simulink model "HCS_Sim_r9_final"  (R2023a)
settings: Solver=ode4  StartTime=0.0  StopTime=24  FixedStep=5e-3  RelTol=1e-3  EnableMultiTasking=on
libraries: simulink x26, simulink_extras x11, arduinolib x8, spspowerguiLib x1
(part 1 of 5)
settings Model: ExtModeTrigDuration=2  Creator=jakob  LastModifiedBy=Matt Smith
settings OptimizationCC: EnhancedBackFolding=on  PassReuseOutputArgsAs=Individual arguments  ZeroExternalMemoryAtStartup=off  ZeroInternalMemoryAtStartup=off  MaxStackSize=64  OptimizeBlockOrder=speed  DifferentSizesBufferReuse=on  OptimizationCustomize=off  EfficientTunableParamExpr=on
settings DebuggingCC: ParameterTunabilityLossMsg=error  UnderSpecifiedDimensionMsg=warning
settings HardwareCC: ProdBitPerInt=16  ProdBitPerPointer=16  ProdBitPerSizeT=16  ProdBitPerPtrDiffT=16  ProdLargestAtomicFloat=None  ProdWordSize=8  ProdHWDeviceType=Atmel->AVR
settings SFSimCC: MATLABDynamicMemAlloc=off  SimTargetLang=C++
settings RTWCC: Description=Embedded Coder  SystemTargetFile=ert.tlc  HardwareBoard=Arduino Uno  TemplateMakefile=ert_default_tmf  Toolchain=Arduino AVR  BuildConfiguration=Faster Runs
settings CodeAppCC: ForceParamTrailComments=on  IgnoreCustomStorageClasses=off  OperatorAnnotations=on  SimulinkDataObjDesc=on  SFDataObjDesc=on  InsertBlockDesc=on
settings ERTTargetCC: SupportContinuousTime=on  SupportVariableSizeSignals=on  ExtModeTransport=3  ExtModeStaticAlloc=on  ExtModeAutomaticAllocSize=off  ExtModeStaticAllocSize=250  ExtModeMexFile=ext_xcp  ExtModeIntrfLevel=Level2 - Open

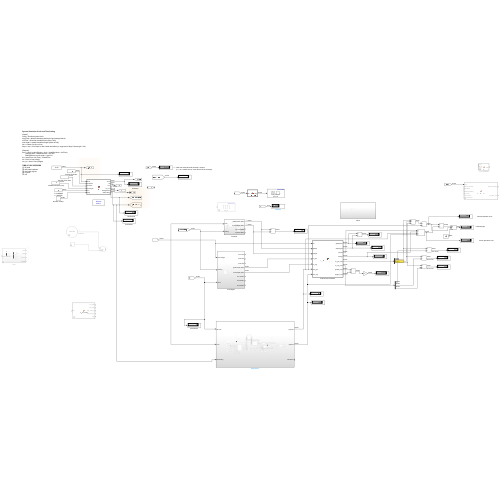
[thumbnail: Simulink's stored preview of the top-level diagram]
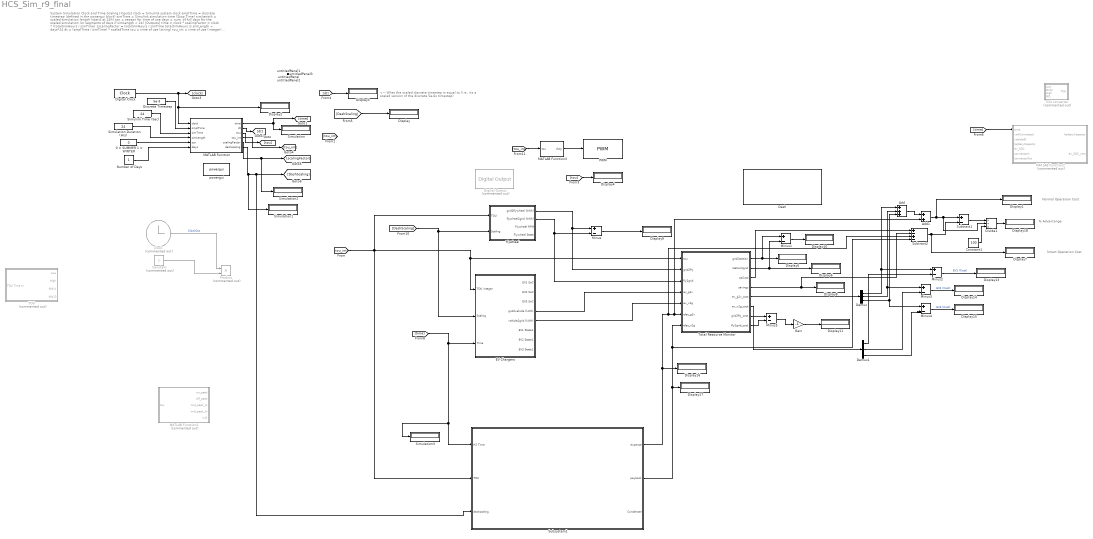
== system HCS_Sim_r9_final ==
  note: Smart Operation Cost
  note: % Advantange
  note: Normal Operation Cost
  note: <--- What the scaled discrete timestep is equal to
      | 	(i.e., its a scaled version of the discrete 5e-6s timestep)
  note: System Simulation Clock and Time Scaling
      |
      | [Inputs]
      | clock = Simulink system clock
      | smplTime = discrete timestep (defined in the powergui block)
      | simTime = Simulink simulation time (Stop Time)
      | simLength = scaled simulation length (static at 24h)
      | szn = season for time of use
      | days = num. of full days for the scaled simulation (or segments of days if simLength < 24)
      |
      | [Outputs]
      | time = clock * scalingFactor = clock * (totalSimHours / simTime)
      | {scalingFactor = totalSimHours / simTime
      | totalSimHours is simLength + days*24
      | dt = (smplTime / simTime) * scaledTime
      | tou = time of use (string)
      | tou_int = time of use (integer)
      |
      | TIME OF USE INTEGERS
      | [1] off peak
      | [2] mid peak low/down
      | [3] mid peak high/up
      | [4] on peak
      | [5] null
  0 = SUMMER 1 = WINTER : Constant  Value=0
  Add : Sum  Inputs=+++
  Add1 : Sum
  Clock : Clock  Commented=on
  Constant : Constant  Commented=on
  Constant1 : Constant  Value=100
  Dash : Subsystem
  Demux : Demux  Outputs=3
  Demux1 : Demux  Outputs=3
  Digital Clock : DigitalClock  SampleTime=5e-3
  Digital Output : arduinolib/Digital Output  Commented=on  pinNumber=9  Direction=output  blockPlatform=arduino
  Discrete Timestep : Constant  Value=5e-3
  Display{,1..11,13..18} (18 alike) : Display
  Divide1 : Product  Inputs=*/*
  EV Chargers : Subsystem
  Flywheel : Subsystem  StopFcn=CapTest
  Gain : Gain  Gain=-1
  MATLAB Function : MATLAB Function  TreatAsAtomicUnit=on
  MATLAB Function1 : MATLAB Function  Commented=on  TreatAsAtomicUnit=on
  MATLAB Function2 : MATLAB Function  Commented=on  TreatAsAtomicUnit=on
  MATLAB Function3 : MATLAB Function  TreatAsAtomicUnit=on
  Minus{,1..5} (6 alike) : Sum  Inputs=+-
  Number of Days : Constant
  PWM : arduinolib/PWM  pinNumber=10  frequencyType=Default  desiredFrequency=490.2  achievableFrequency=490.1961
  Product : Product  Commented=on
  Simulation{,1..3} (4 alike) : Display
  Simulation Duration (Hrs) : Constant  Value=24
  Simulink Time (Sec) : Constant  Value=24
  Subsystem1 : Subsystem
  Subtract1 : Sum  Inputs=+-
  Subtract2 : Sum  Inputs=+-+-
  TOU : Subsystem  Commented=on
  TOU converter : MATLAB Function  Commented=on  TreatAsAtomicUnit=on
  Total Resource Monitor : MATLAB Function  TreatAsAtomicUnit=on
  powergui : spspowerguiLib/powergui  Priority=1  SimulationMode=Discrete  SampleTime=5e-3  frequency=60  Iterations=50  frequencyindice=0  Pbase=100e6  ErrMax=1e-4  UnitsV=kV  UnitsW=MW  buscounter=0  FunctionMessages=off  echomessages=off  EnableUseOfTLC=off  CurrentSourceSwitches=off  DisableSnubberDevices=off  DisableRonSwitches=off  DisableVfSwitches=off  DisplayEquations=off  AutomaticDiscreteSolvers=off  SolverType=Tustin/Backward Euler (TBE)  Interpol=off  ExternalGateDelay=off  methode=off  Ts=100  x0status=blocks  SPID=on  SwTol=0  HookPort=off  NonlinearTolerance=1e-4  nMaxIteration=100  ContinueOnMaxIteration=off  RestoreLinks=warning  ResistiveCurrentMeasurement=off  Frange=[0:2:500]  Ylog=off  Xlog=on  ShowGrid=off  save=off  variable=ZData  structure=0  ZoomFFT=off  StartTime=0.0  cycles=1  DisplayStyle=1  fundamental=60  FreqAxis=off  MaxFrequency=1000  frequencyindicesteady=1  RmsSteady=1  display=off
  untitledPanel : Subsystem  Tag=HiddenForWebPanel  IsWebBlockPanel=on
  untitledPanel1 : Subsystem  Tag=HiddenForWebPanel  IsWebBlockPanel=on
  untitledPanel2 : Subsystem  Tag=HiddenForWebPanel  IsWebBlockPanel=on
  untitledPanel3 : Subsystem  Tag=HiddenForWebPanel  IsWebBlockPanel=on
  wires:
  Clock/1 -> Product/1  "ClockOut"
  Constant/1 -> Product/2
  MATLAB Function/1(time) -> [time], Simulation/1
  MATLAB Function/3(tou) -> [tou]
  Digital Clock/1 -> [clock], MATLAB Function/1(clock), Display2/1
  Number of Days/1 -> MATLAB Function/6(days)
  Discrete Timestep/1 -> MATLAB Function/2(smplTime)
  Simulink Time (Sec)/1 -> MATLAB Function/3(simTime)
  Simulation Duration (Hrs)/1 -> MATLAB Function/4(simLength)
  MATLAB Function/4(tou_int) -> [tou_int]
  MATLAB Function/2(dt) -> [dt]
  0 = SUMMER 1 = WINTER/1 -> MATLAB Function/5(szn)
  [tou] -> Display4/1
  [dt] -> Display3/1
  MATLAB Function/5(scalingFactor) -> Simulation2/1, [scalingFactor]
  [tou_int] -> Subsystem1/2(TOU), EV Chargers/1(TOU integer), Total Resource Monitor/1(tou), Flywheel/1(TOU)
  [time] -> MATLAB Function2/1(time)
  MATLAB Function/6(dashscaling) -> Simulation1/1, Subsystem1/3(dashscaling), [DashScaling]
  [DashScaling] -> Display/1
  [tou_int] -> MATLAB Function3/1(tou)
  MATLAB Function3/1(duty) -> PWM/1
  [DashScaling] -> Flywheel/2(Scaling), EV Chargers/2(Scaling)
  Flywheel/1(grid2flywheel (kWh)) -> Total Resource Monitor/2(grid2fly), Minus/1
  Flywheel/2(flywheel2grid (kWh)) -> Total Resource Monitor/3(fly2grid), Minus/2
  Total Resource Monitor/1(grid2station) -> Minus1/1, Display5/1
  Total Resource Monitor/2(station2grid) -> Minus1/2, Display6/1
  Total Resource Monitor/3(opCost) -> Subtract2/1
  Total Resource Monitor/4(savings) -> Subtract2/2, Display8/1
  Total Resource Monitor/5(ev_g2v_cost) -> Demux/1
  [time] -> Subsystem1/1(H2 Time), Simulation3/1, EV Chargers/3(Time)
  Total Resource Monitor/7(grid2fly_cost) -> Minus5/1
  Total Resource Monitor/8(fly2grid_cost) -> Minus5/2
  EV Chargers/4(grid2vehicle (kWh)) -> Total Resource Monitor/4(ev_g2v)
  EV Chargers/5(vehicle2grid (kWh)) -> Total Resource Monitor/5(ev_v2g)
  Demux1/3 -> Minus4/2
  Total Resource Monitor/6(ev_v2g_cost) -> Demux1/1
  Demux1/2 -> Minus3/2
  Demux1/1 -> Minus2/2
  Demux/3 -> Minus4/1, Add/3
  Demux/2 -> Add/2, Minus3/1
  Demux/1 -> Add/1, Minus2/1
  Minus/1 -> Display9/1
  Minus1/1 -> Display10/1
  Minus2/1 -> Display13/1  "EV1 (Cost)"
  Minus3/1 -> Display14/1  "EV2 (Cost)"
  Minus4/1 -> Display15/1  "EV3 (Cost)"
  Minus5/1 -> Gain/1
  Gain/1 -> Display11/1
  Subsystem1/2(payback) -> Display17/1, Subtract2/4, Total Resource Monitor/7(elec_v2g)
  Subsystem1/1(expense) -> Display16/1, Subtract2/3, Add1/2, Total Resource Monitor/6(elec_g2v)
  Add/1 -> Add1/1
  Add1/1 -> Display1/1, Divide1/2, Subtract1/1
  Subtract2/1 -> Display7/1, Subtract1/2
  Subtract1/1 -> Divide1/1
  Divide1/1 -> Display18/1
  Constant1/1 -> Divide1/3

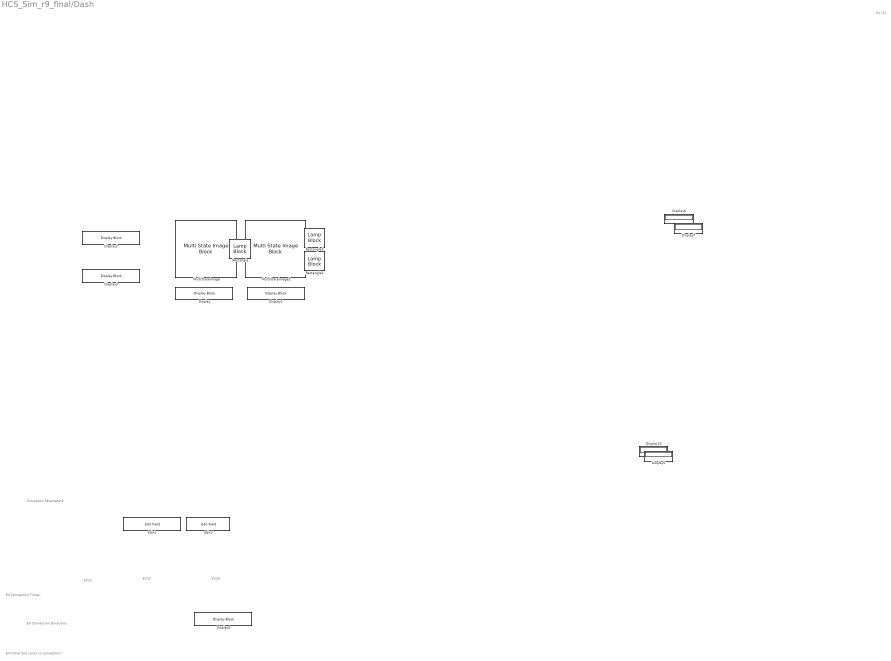
== system HCS_Sim_r9_final/Dash ==
  note: EV (2)
  note: EV Connection Times:
  note: EV Connection
      | Durations:
  note: EV Initial SoC (prior
      | to connection):
  note: EV(1)
  note: EV(2)
  note: EV(3)
  note: Simulation Parameters:
  Display{,1..4} (5 alike) : DisplayBlock  LabelPosition=Hide  Transparency=1
      Display2 settings: AttributesFormatString=Hydrogen Output (KG)
      Display3 settings: AttributesFormatString=FCEVs Fueled
  Display{5..7,16} (4 alike) : Display
  Edit1 : EditField  LabelPosition=Bottom  ShowInitialText=on  Alignment=Center
  Edit2 : EditField  LabelPosition=Bottom  ShowInitialText=on  Alignment=Center
  MultiStateImage : MultiStateImageBlock  Description=10KG pressurized 700Bar
      settings: AttributesFormatString=10KG pressurized 700Bar
  MultiStateImage1 : MultiStateImageBlock
      settings: AttributesFormatString=10KG pressurized 200Bar
  Rectangle : LampBlock  LabelPosition=Hide  Icon=Rectangle
      settings: AttributesFormatString=Compressor
  Rectangle2 : LampBlock  LabelPosition=Hide  Icon=Rectangle
      settings: AttributesFormatString=Reverse Electrolysis
  Rectangle3 : LampBlock  LabelPosition=Hide  Icon=Rectangle
      settings: AttributesFormatString=Electrolysis

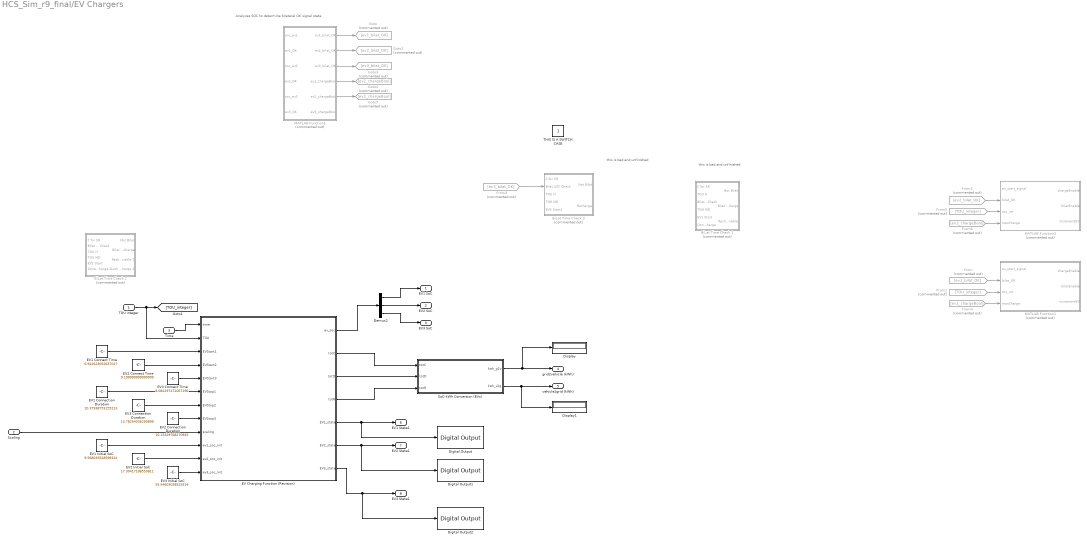
== system HCS_Sim_r9_final/EV Chargers ==
  note: this is bad and unfinished
  note: Analyzes SOC to determine bilateral OK signal state
  note: this is bad and unfinished
  TOU integer : Inport
  Scaling : Inport  Port=2
  Time : Inport  Port=3
  BiLat Time Check 1 : Subsystem  Commented=on
  BiLat Time Check 2 : Subsystem  Commented=on
  BiLat Time Check 3 : Subsystem  Commented=on
  Demux2 : Demux  Outputs=3
  Digital Output : arduinolib/Digital Output  pinNumber=6  Direction=output  blockPlatform=arduino
  Digital Output1 : arduinolib/Digital Output  pinNumber=7  Direction=output  blockPlatform=arduino
  Digital Output2 : arduinolib/Digital Output  pinNumber=8  Direction=output  blockPlatform=arduino
  Display : Display
  Display1 : Display
  EV Charging Function (Revision) : MATLAB Function  TreatAsAtomicUnit=on
  EV1 Connect Time : Constant  Value=6.922623052637027
  EV1 Connection Duration : Constant  Value=10.37938753155213
  EV1 Initial SoC : Constant  Value=9.568033528599324
  EV2 Connect Time : Constant  Value=9.199999999999999
  EV2 Connection Duration : Constant  Value=10.15329768270945
  EV2 Initial SoC : Constant  Value=17.30417188553811
  EV3 Connect Time : Constant  Value=8.082297471067296
  EV3 Connection Duration : Constant  Value=13.78254036290899
  EV3 Initial SoC : Constant  Value=55.54603038529314
  From : From  Commented=on  GotoTag=ev1_bilat_OK
  From1 : From  Commented=on  GotoTag=TOU_integer
  From2 : From  Commented=on  GotoTag=ev2_bilat_OK
  From3 : From  Commented=on  GotoTag=ev3_bilat_OK
  From4 : From  Commented=on  GotoTag=ev1_chargeBool
  From5 : From  Commented=on  GotoTag=TOU_integer
  From6 : From  Commented=on  GotoTag=ev2_chargeBool
  Goto : Goto  Commented=on  GotoTag=ev1_bilat_OK
  Goto2 : Goto  Commented=on  GotoTag=ev2_bilat_OK
  Goto3 : Goto  Commented=on  GotoTag=ev3_bilat_OK
  Goto4 : Goto  Commented=on  GotoTag=ev1_chargeBool
  Goto5 : Goto  Commented=on  GotoTag=ev2_chargeBool
  MATLAB Function1 : MATLAB Function  Commented=on  TreatAsAtomicUnit=on
  MATLAB Function2 : MATLAB Function  Commented=on  TreatAsAtomicUnit=on
  MATLAB Function3 : MATLAB Function  Commented=on  TreatAsAtomicUnit=on
  SoC-kWh Conversion (EVs) : MATLAB Function  TreatAsAtomicUnit=on
  THIS IS A SWITCH CASE : Constant
  EV1 SoC : Outport
  EV2 SoC : Outport  Port=2
  EV3 SoC : Outport  Port=3
  grid2vehicle (kWh) : Outport  Port=4
  vehicle2grid (kWh) : Outport  Port=5
  EV1 State1 : Outport  Port=6
  EV2 State1 : Outport  Port=7
  EV3 State1 : Outport  Port=8
  wires:
  MATLAB Function1/1(ev1_bilat_OK) -> Goto/1
  MATLAB Function1/2(ev2_bilat_OK) -> Goto2/1
  MATLAB Function1/3(ev3_bilat_OK) -> Goto3/1
  From/1 -> MATLAB Function2/2(bilat_OK)
  From1/1 -> MATLAB Function2/3(tou_int)
  From3/1 -> BiLat Time Check 3/2(Bilat SOC Check)
  MATLAB Function1/4(ev1_chargeBool) -> Goto4/1
  From4/1 -> MATLAB Function2/4(maxCharge)
  From2/1 -> MATLAB Function3/2(bilat_OK)
  From5/1 -> MATLAB Function3/3(tou_int)
  From6/1 -> MATLAB Function3/4(maxCharge)
  MATLAB Function1/5(ev2_chargeBool) -> Goto5/1
  Scaling/1 -> EV Charging Function (Revision)/9(scaling)
  TOU integer/1 -> EV Charging Function (Revision)/2(TOU), [TOU_integer]
  SoC-kWh Conversion (EVs)/1(kwh_g2v) -> Display/1, grid2vehicle (kWh)/1
  SoC-kWh Conversion (EVs)/2(kwh_v2g) -> Display1/1, vehicle2grid (kWh)/1
  Time/1 -> EV Charging Function (Revision)/1(time)
  EV3 Connect Time/1 -> EV Charging Function (Revision)/5(EVStart3)
  EV2 Connect Time/1 -> EV Charging Function (Revision)/4(EVStart2)
  EV1 Connect Time/1 -> EV Charging Function (Revision)/3(EVStart1)
  EV2 Connection Duration/1 -> EV Charging Function (Revision)/8(EVStop3)
  EV3 Connection Duration/1 -> EV Charging Function (Revision)/7(EVStop2)
  EV1 Connection Duration/1 -> EV Charging Function (Revision)/6(EVStop1)
  EV Charging Function (Revision)/1(ev_soc) -> Demux2/1
  Demux2/1 -> EV1 SoC/1
  Demux2/2 -> EV2 SoC/1
  Demux2/3 -> EV3 SoC/1
  EV Charging Function (Revision)/2(totC) -> SoC-kWh Conversion (EVs)/1(totC)
  EV Charging Function (Revision)/3(totD) -> SoC-kWh Conversion (EVs)/2(totD)
  EV Charging Function (Revision)/4(totR) -> SoC-kWh Conversion (EVs)/3(totR)
  EV Charging Function (Revision)/5(EV1_state) -> Digital Output/1, EV1 State1/1
  EV Charging Function (Revision)/6(EV2_state) -> Digital Output1/1, EV2 State1/1
  EV Charging Function (Revision)/7(EV3_state) -> Digital Output2/1, EV3 State1/1
  EV1 Initial SoC/1 -> EV Charging Function (Revision)/10(ev1_soc_init)
  EV2 Initial SoC/1 -> EV Charging Function (Revision)/11(ev2_soc_init)
  EV3 Initial SoC/1 -> EV Charging Function (Revision)/12(ev3_soc_init)

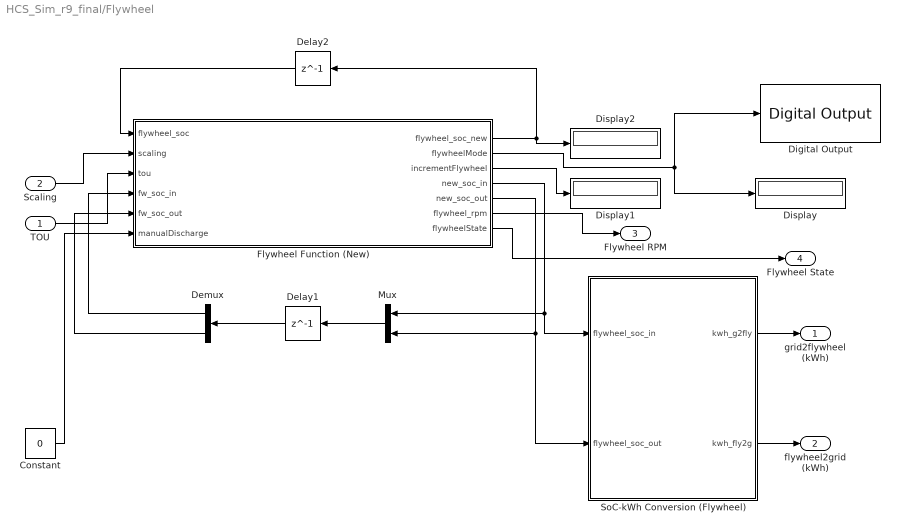
== system HCS_Sim_r9_final/Flywheel ==
  TOU : Inport
  Scaling : Inport  Port=2
  Constant : Constant  Value=0
  Delay1 : Delay  DelayLength=1
  Delay2 : Delay  DelayLength=1
  Demux : Demux  Outputs=2
  Digital Output : arduinolib/Digital Output  pinNumber=5  Direction=output  blockPlatform=arduino
  Display : Display
      settings: Decimation=4
  Display1 : Display
      settings: Decimation=4
  Display2 : Display
      settings: Decimation=4
  Flywheel Function (New) : MATLAB Function  TreatAsAtomicUnit=on
  Mux : Mux  Inputs=2
  SoC-kWh Conversion (Flywheel) : MATLAB Function  TreatAsAtomicUnit=on
  grid2flywheel (kWh) : Outport
  flywheel2grid (kWh) : Outport  Port=2
  Flywheel RPM : Outport  Port=3
  Flywheel State : Outport  Port=4
  wires:
  Flywheel Function (New)/1(flywheel_soc_new) -> Delay2/1, Display2/1
  Delay2/1 -> Flywheel Function (New)/1(flywheel_soc)
  Scaling/1 -> Flywheel Function (New)/2(scaling)
  TOU/1 -> Flywheel Function (New)/3(tou)
  Flywheel Function (New)/3(incrementFlywheel) -> Display1/1
  Flywheel Function (New)/2(flywheelMode) -> Display/1, Digital Output/1
  SoC-kWh Conversion (Flywheel)/1(kwh_g2fly) -> grid2flywheel (kWh)/1
  SoC-kWh Conversion (Flywheel)/2(kwh_fly2g) -> flywheel2grid (kWh)/1
  Mux/1 -> Delay1/1
  Flywheel Function (New)/4(new_soc_in) -> SoC-kWh Conversion (Flywheel)/1(flywheel_soc_in), Mux/1
  Flywheel Function (New)/5(new_soc_out) -> Mux/2, SoC-kWh Conversion (Flywheel)/2(flywheel_soc_out)
  Delay1/1 -> Demux/1
  Demux/1 -> Flywheel Function (New)/4(fw_soc_in)
  Demux/2 -> Flywheel Function (New)/5(fw_soc_out)
  Flywheel Function (New)/6(flywheel_rpm) -> Flywheel RPM/1
  Flywheel Function (New)/7(flywheelState) -> Flywheel State/1
  Constant/1 -> Flywheel Function (New)/6(manualDischarge)

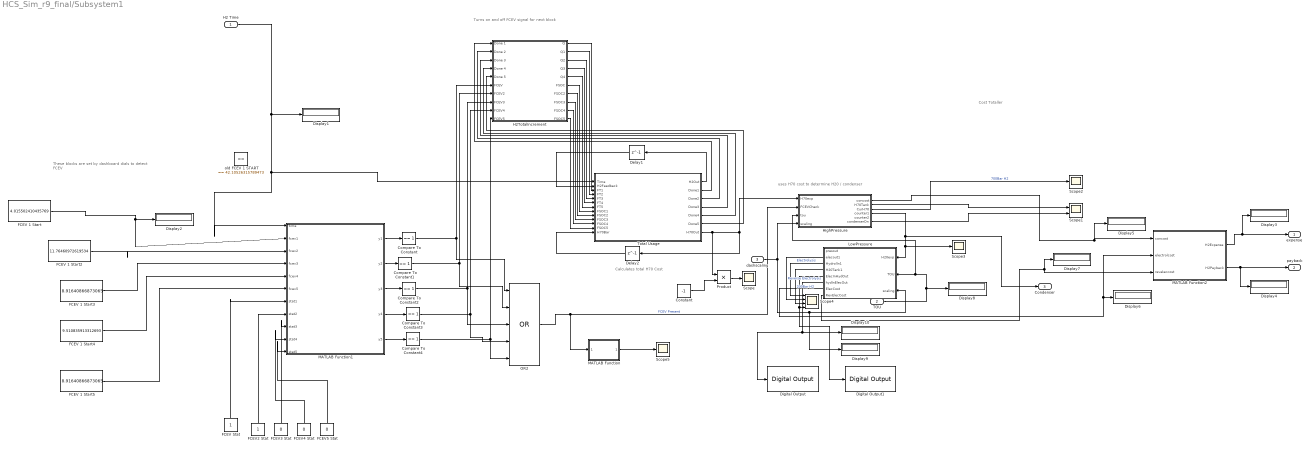
== system HCS_Sim_r9_final/Subsystem1 ==
  note: uses H70 cost to determine H20 / condenser
  note: Calculates total H70 Cost
  note: Turns on and off FCEV signal for next block
  note: These blocks are set by dashboard dials to detect FCEV
  note: Cost Totaller
  H2 Time : Inport
  TOU : Inport  Port=2
  dashscaling : Inport  Port=3
  Compare To Constant{,1..4} (5 alike) : simulink/Logic and Bit Operations/Compare To Constant  relop===  const=1  OutDataTypeStr=boolean
  Constant : Constant  Value=-1
  Delay1 : Delay  DelayLength=1  InitialCondition=0
  Delay2 : Delay  DelayLength=1  InitialCondition=0
  Digital Output : arduinolib/Digital Output  pinNumber=4  Direction=output  blockPlatform=arduino
  Digital Output1 : arduinolib/Digital Output  pinNumber=3  Direction=output  blockPlatform=arduino
  Display{1..10} (10 alike) : Display
  FCEV 1 Start : Constant  Value=4.015502410435769
  FCEV 1 Start2 : Constant  Value=11.76460972619534
  FCEV 1 Start3 : Constant  Value=8.91640866873065
  FCEV 1 Start4 : Constant  Value=9.510835913312693
  FCEV 1 Start5 : Constant  Value=8.91640866873065
  FCEV Stat : Constant
  FCEV2 Stat : Constant
  FCEV3 Stat : Constant  Value=0
  FCEV4 Stat : Constant  Value=0
  FCEV5 Stat : Constant  Value=0
  H2TotalIncrement : Subsystem
  HighPressure : MATLAB Function  TreatAsAtomicUnit=on
  LowPressure : MATLAB Function  TreatAsAtomicUnit=on
  MATLAB Function : MATLAB Function  TreatAsAtomicUnit=on
  MATLAB Function1 : MATLAB Function  TreatAsAtomicUnit=on
  MATLAB Function2 : MATLAB Function  TreatAsAtomicUnit=on
  OR2 : Logic  Operator=OR  Inputs=5  IconShape=distinctive  AllPortsSameDT=off  OutDataTypeStr=boolean
  Product : Product
  Scope{,2..3,5} (4 alike) : Scope
  Scope1 : Scope  NumInputPorts=2
  Scope4 : Scope  NumInputPorts=4
  Total Usage : MATLAB Function  TreatAsAtomicUnit=on
  old FCEV 1 START : simulink/Logic and Bit Operations/Compare To Constant  relop===  const=42.10526315789473  OutDataTypeStr=boolean
  expense : Outport
  payback : Outport  Port=2
  Condenser : Outport  Port=3
  wires:
  MATLAB Function1/1(y1) -> Compare To Constant/1
  OR2/1 -> MATLAB Function/1(FCEVIn), HighPressure/2(FCEVCheck)  "FCEV Present"
  MATLAB Function1/3(y3) -> Compare To Constant2/1
  MATLAB Function1/2(y2) -> Compare To Constant1/1
  Total Usage/1(H2Out) -> Delay1/1
  MATLAB Function1/4(y4) -> Compare To Constant3/1
  MATLAB Function1/5(y5) -> Compare To Constant4/1
  Total Usage/2(Done1) -> H2TotalIncrement/1(Done 1)
  Total Usage/3(Done2) -> H2TotalIncrement/2(Done 2)
  Total Usage/4(Done3) -> H2TotalIncrement/3(Done 3)
  Total Usage/5(Done4) -> H2TotalIncrement/4(Done 4)
  Total Usage/6(Done5) -> H2TotalIncrement/5(Done 5)
  Total Usage/7(H70Out) -> Product/1, Delay2/1, HighPressure/1(H70exp)
  H2TotalIncrement/1(Q) -> Total Usage/3(FT1)
  H2TotalIncrement/2(Q1) -> Total Usage/4(FT2)
  H2TotalIncrement/3(Q2) -> Total Usage/5(FT3)
  H2TotalIncrement/4(Q3) -> Total Usage/6(FT4)
  H2TotalIncrement/5(Q4) -> Total Usage/7(FT5)
  Delay2/1 -> Total Usage/13(H70Bar)
  H2TotalIncrement/6(FSOC) -> Total Usage/8(FSOC1)
  H2TotalIncrement/7(FSOC2) -> Total Usage/9(FSOC2)
  H2TotalIncrement/8(FSOC3) -> Total Usage/10(FSOC3)
  H2TotalIncrement/9(FSOC4) -> Total Usage/11(FSOC4)
  H2TotalIncrement/10(FSOC5) -> Total Usage/12(FSOC5)
  Delay1/1 -> Total Usage/2(H2Feedback)
  HighPressure/2(H70Tank) -> Scope1/1
  HighPressure/3(CurH70) -> Scope2/1  "700Bar H2"
  HighPressure/4(counter1) -> Condenser/1, LowPressure/1(H20exp), Scope3/1
  TOU/1 -> Display8/1, HighPressure/3(tou), LowPressure/2(TOU)
  LowPressure/3(HydrolIn1) -> Scope4/1  "Electrolysis"
  LowPressure/2(elecout1) -> Scope4/2  "Reverse Electrolysis"
  LowPressure/4(H20Tank1) -> Scope4/3  "200Bar H2"
  LowPressure/5(ElecInHydOut) -> Digital Output1/1, Scope4/4
  HighPressure/6(condenserOn) -> Scope1/2
  MATLAB Function/1(FCEVPres) -> Scope5/1
  FCEV 1 Start/1 -> MATLAB Function1/2(fcev1), Display2/1
  FCEV Stat/1 -> MATLAB Function1/7(stat1)
  FCEV2 Stat/1 -> MATLAB Function1/8(stat2)
  FCEV3 Stat/1 -> MATLAB Function1/9(stat3)
  FCEV4 Stat/1 -> MATLAB Function1/10(stat4)
  FCEV5 Stat/1 -> MATLAB Function1/11(stat5)
  FCEV 1 Start5/1 -> MATLAB Function1/6(fcev5)
  FCEV 1 Start4/1 -> MATLAB Function1/5(fcev4)
  FCEV 1 Start3/1 -> MATLAB Function1/4(fcev3)
  FCEV 1 Start2/1 -> MATLAB Function1/3(fcev2)
  Compare To Constant/1 -> H2TotalIncrement/6(FCEV), OR2/1
  Compare To Constant1/1 -> H2TotalIncrement/7(FCEV2), OR2/2
  Compare To Constant2/1 -> H2TotalIncrement/8(FCEV3), OR2/3
  Compare To Constant3/1 -> H2TotalIncrement/9(FCEV4), OR2/4
  Compare To Constant4/1 -> H2TotalIncrement/10(FCEV5), OR2/5
  H2 Time/1 -> Display1/1, MATLAB Function1/1(time), Total Usage/1(Time)
  Constant/1 -> Product/2
  Product/1 -> Scope/1
  HighPressure/1(concost) -> Display5/1, MATLAB Function2/1(concost)
  dashscaling/1 -> HighPressure/4(scaling), Display9/1, LowPressure/3(scaling)
  MATLAB Function2/1(H2Expense) -> Display3/1, expense/1
  MATLAB Function2/2(H2Payback) -> Display4/1, payback/1
  LowPressure/7(ElecCost) -> Display6/1, MATLAB Function2/2(electrolcost)
  LowPressure/8(RevElecCost) -> Display7/1, MATLAB Function2/3(reveleccost)
  LowPressure/6(hydInElecOut) -> Display10/1, Digital Output/1

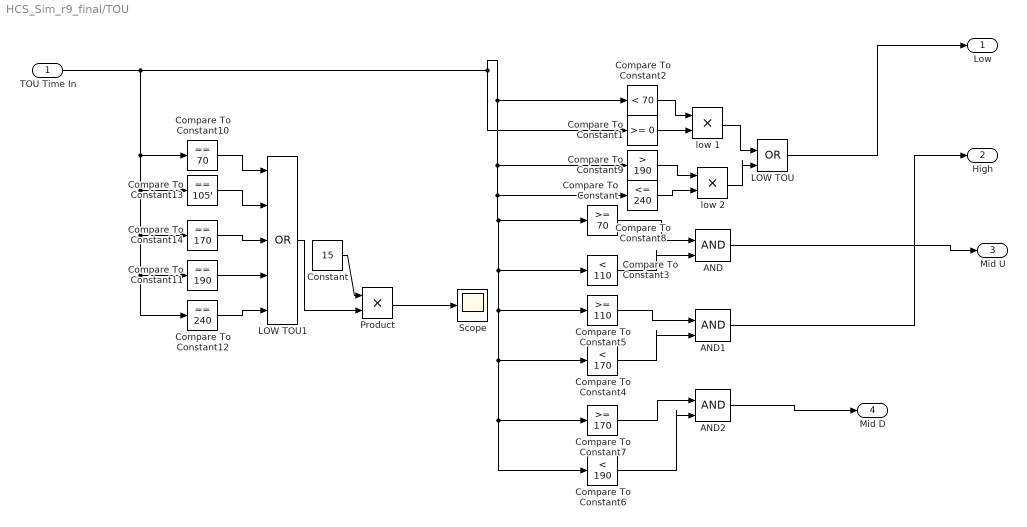
== system HCS_Sim_r9_final/TOU ==
  TOU Time In : Inport
  AND : Logic  IconShape=distinctive  AllPortsSameDT=off  OutDataTypeStr=boolean
  AND1 : Logic  IconShape=distinctive  AllPortsSameDT=off  OutDataTypeStr=boolean
  AND2 : Logic  IconShape=distinctive  AllPortsSameDT=off  OutDataTypeStr=boolean
  Compare To Constant : simulink/Logic and Bit Operations/Compare To Constant  relop=>=  const=70  OutDataTypeStr=boolean
  Compare To Constant1 : simulink/Logic and Bit Operations/Compare To Constant  relop=>=  const=0  OutDataTypeStr=boolean
  Compare To Constant10 : simulink/Logic and Bit Operations/Compare To Constant  relop===  const=70  OutDataTypeStr=boolean
  Compare To Constant11 : simulink/Logic and Bit Operations/Compare To Constant  relop===  const=190  OutDataTypeStr=boolean
  Compare To Constant12 : simulink/Logic and Bit Operations/Compare To Constant  relop===  const=240  OutDataTypeStr=boolean
  Compare To Constant13 : simulink/Logic and Bit Operations/Compare To Constant  relop===  const=105'  OutDataTypeStr=boolean
  Compare To Constant14 : simulink/Logic and Bit Operations/Compare To Constant  relop===  const=170  OutDataTypeStr=boolean
  Compare To Constant2 : simulink/Logic and Bit Operations/Compare To Constant  relop=<  const=70  OutDataTypeStr=boolean
  Compare To Constant3 : simulink/Logic and Bit Operations/Compare To Constant  relop=<  const=110  OutDataTypeStr=boolean
  Compare To Constant4 : simulink/Logic and Bit Operations/Compare To Constant  relop=<  const=170  OutDataTypeStr=boolean
  Compare To Constant5 : simulink/Logic and Bit Operations/Compare To Constant  relop=>=  const=110  OutDataTypeStr=boolean
  Compare To Constant6 : simulink/Logic and Bit Operations/Compare To Constant  relop=<  const=190  OutDataTypeStr=boolean
  Compare To Constant7 : simulink/Logic and Bit Operations/Compare To Constant  relop=>=  const=170  OutDataTypeStr=boolean
  Compare To Constant8 : simulink/Logic and Bit Operations/Compare To Constant  relop=<=  const=240  OutDataTypeStr=boolean
  Compare To Constant9 : simulink/Logic and Bit Operations/Compare To Constant  relop=>  const=190  OutDataTypeStr=boolean
  Constant : Constant  Value=15
  LOW TOU : Logic  Operator=OR  IconShape=distinctive  AllPortsSameDT=off  OutDataTypeStr=boolean
  LOW TOU1 : Logic  Operator=OR  Inputs=5  IconShape=distinctive  AllPortsSameDT=off  OutDataTypeStr=boolean
  Product : Product
  Scope : Scope
  low 1 : Product
  low 2 : Product
  Low : Outport
  High : Outport  Port=2
  Mid U : Outport  Port=3
  Mid D : Outport  Port=4
  wires:
  Compare To Constant6/1 -> AND2/2
  Compare To Constant/1 -> AND/1
  low 2/1 -> LOW TOU/2
  Compare To Constant5/1 -> AND1/1
  Compare To Constant8/1 -> low 2/2
  TOU Time In/1 -> Compare To Constant12/1, Compare To Constant11/1, Compare To Constant14/1, Compare To Constant13/1, Compare To Constant10/1, Compare To Constant9/1, Compare To Constant8/1, Compare To Constant6/1, Compare To Constant7/1, Compare To Constant4/1, Compare To Constant5/1, Compare To Constant3/1, Compare To Constant/1, Compare To Constant2/1, Compare To Constant1/1
  Compare To Constant3/1 -> AND/2
  AND1/1 -> High/1
  Compare To Constant2/1 -> low 1/1
  Compare To Constant1/1 -> low 1/2
  Compare To Constant7/1 -> AND2/1
  Compare To Constant4/1 -> AND1/2
  AND/1 -> Mid U/1
  Compare To Constant9/1 -> low 2/1
  low 1/1 -> LOW TOU/1
  LOW TOU/1 -> Low/1
  AND2/1 -> Mid D/1
  Constant/1 -> Product/1
  LOW TOU1/1 -> Product/2
  Product/1 -> Scope/1
  Compare To Constant10/1 -> LOW TOU1/1
  Compare To Constant13/1 -> LOW TOU1/2
  Compare To Constant14/1 -> LOW TOU1/3
  Compare To Constant11/1 -> LOW TOU1/4
  Compare To Constant12/1 -> LOW TOU1/5

== system HCS_Sim_r9_final/untitledPanel ==
  Slider Switch : SliderSwitchBlock  Tag=HiddenForWebPanel  PanelInfo="{\"height\":67,\"left\":756,\"panelId\":\"panelId-6772c4c8-0595-4f8c-93bd-17566f64b2d4\",\"top\":63,\"type\":\"panelChild\",\"version\":\"2019b\",\"width\":270,\"zIndex\":1500026}"  LabelPosition=Hide
      settings: Values={{'Summer TOU', 'Winter TOU'}, [0 1]}
  Slider10 : SliderBlock  Tag=HiddenForWebPanel  PanelInfo="{\"height\":168,\"left\":822,\"panelId\":\"panelId-6772c4c8-0595-4f8c-93bd-17566f64b2d4\",\"top\":181,\"type\":\"panelChild\",\"version\":\"2019b\",\"width\":375,\"zIndex\":1500008}"  LabelPosition=Hide  ScaleMax=24  TickInterval=2
  Slider11 : SliderBlock  Tag=HiddenForWebPanel  PanelInfo="{\"height\":168,\"left\":44,\"panelId\":\"panelId-6772c4c8-0595-4f8c-93bd-17566f64b2d4\",\"top\":471,\"type\":\"panelChild\",\"version\":\"2019b\",\"width\":375,\"zIndex\":1500004}"  LabelPosition=Hide
  Slider12 : SliderBlock  Tag=HiddenForWebPanel  PanelInfo="{\"height\":168,\"left\":422,\"panelId\":\"panelId-6772c4c8-0595-4f8c-93bd-17566f64b2d4\",\"top\":475,\"type\":\"panelChild\",\"version\":\"2019b\",\"width\":371,\"zIndex\":1500020}"  LabelPosition=Hide  TickInterval=10
  Slider13 : SliderBlock  Tag=HiddenForWebPanel  PanelInfo="{\"height\":168,\"left\":811,\"panelId\":\"panelId-6772c4c8-0595-4f8c-93bd-17566f64b2d4\",\"top\":471,\"type\":\"panelChild\",\"version\":\"2019b\",\"width\":375,\"zIndex\":1500002}"  LabelPosition=Hide  TickInterval=10
  Slider5 : SliderBlock  Tag=HiddenForWebPanel  PanelInfo="{\"height\":168,\"left\":50,\"panelId\":\"panelId-6772c4c8-0595-4f8c-93bd-17566f64b2d4\",\"top\":319,\"type\":\"panelChild\",\"version\":\"2019b\",\"width\":375,\"zIndex\":1500022}"  LabelPosition=Hide  ScaleMax=16
  Slider6 : SliderBlock  Tag=HiddenForWebPanel  PanelInfo="{\"height\":168,\"left\":412,\"panelId\":\"panelId-6772c4c8-0595-4f8c-93bd-17566f64b2d4\",\"top\":319,\"type\":\"panelChild\",\"version\":\"2019b\",\"width\":371,\"zIndex\":1500016}"  LabelPosition=Hide  ScaleMax=16
  Slider7 : SliderBlock  Tag=HiddenForWebPanel  PanelInfo="{\"height\":196,\"left\":62,\"panelId\":\"panelId-6772c4c8-0595-4f8c-93bd-17566f64b2d4\",\"top\":171,\"type\":\"panelChild\",\"version\":\"2019b\",\"width\":348,\"zIndex\":1500024}"  LabelPosition=Hide  ScaleMax=24  TickInterval=2
  Slider8 : SliderBlock  Tag=HiddenForWebPanel  PanelInfo="{\"height\":168,\"left\":811,\"panelId\":\"panelId-6772c4c8-0595-4f8c-93bd-17566f64b2d4\",\"top\":314,\"type\":\"panelChild\",\"version\":\"2019b\",\"width\":375,\"zIndex\":1500018}"  LabelPosition=Hide  ScaleMax=16
  Slider9 : SliderBlock  Tag=HiddenForWebPanel  PanelInfo="{\"height\":168,\"left\":419,\"panelId\":\"panelId-6772c4c8-0595-4f8c-93bd-17566f64b2d4\",\"top\":187,\"type\":\"panelChild\",\"version\":\"2019b\",\"width\":371,\"zIndex\":1500000}"  LabelPosition=Hide  ScaleMax=24  TickInterval=2
  panelInfo : PanelWebBlock  Tag=HiddenForWebPanel  PanelInfo="{\"compacted\":false,\"height\":698,\"isActiveTab\":false,\"labels\":{\"label0205069040\":{\"deleted\":false,\"left\":946,\"settings\":{\"backgroundColor\":\"rgba(0, 0, 0, 0)\",\"bold\":true,\"font\":\"Arial\",\"fontColor\":\"black\",\"fontSize\":1.47,\"italicized\":false,\"underlined\":false},\"text\":\"Initial SoC\",\"top\":487},\"label1018222976\":{\"deleted\":false,\"left\":210,\"settings\":{\"backgroundColor\":\"rgba(0, 0, 0, 0)\",\"bold\":true,\"font\":\"Lucida Sans\",\"fontColor\":\"black\",\"fontSize\":1.47,\"italicized\":false,\"underlined\":false},\"text\":\"EV (1)\",\"top\":629},\"label1328676269\":{\"deleted\":false,\"left\":920,\"settings\":{\"backgroundColor\":\"rgba(0, 0, 0, 0)\",\"bold\":true,\"font\":\"Arial\",\"fontColor\":\"black\",\"fontSize\":1.47,\"italicized\":false,\"underlined\":false},\"text\":\"Connection Time\",\"top\":199},\"label2755268504\":{\"deleted\":false,\"left\":504,\"settings\":{\"backgroundColor\":\"rgba(0, 0, 0, 0)\",\"bold\":true,\"font\":\"Lucida Sans\",\"fontColor\":\"black\",\"fontSize\":1.3,\"italicized\":false,\"underlined\":false},\"text\":\"Connection Time \",\"top\":206},\"label3233447872\":{\"deleted\":false,\"left\":147,\"settings\":{\"backgroundColor\":\"rgba(0, 0, 0, 0)\",\"bold\":true,\"font\":\"Lucida Sans\",\"fontColor\":\"black\",\"fontSize\":1.3,\"italicized\":false,\"underlined\":false},\"text\":\"Connection Time\",\"top\":206},\"label4252729118\":{\"deleted\":false,\"left\":172,\"settings\":{\"backgroundColor\":\"rgba(0, 0, 0, 0)\",\"bold\":true,\"font\":\"Arial\",\"fontColor\":\"black\",\"fontSize\":1.47,\"italicized\":false,\"underlined\":false},\"text\":\"Initial SoC\",\"top\":492},\"label4971796399\":{\"deleted\":false,\"left\":580,\"settings\":{\"backgroundColor\":\"rgba(0, 0, 0, 0)\",\"bold\":true,\"font\":\"Lucida Sans\",\"fontColor\":\"black\",\"fontSize\":1.47,\"italicized\":false,\"underlined\":false},\"text\":\"EV (2)\",\"top\":627},\"label5173092740\":{\"deleted\":false,\"left\":973,\"settings\":{\"backgroundColor\":\"rgba(0, 0, 0, 0)\",\"bold\":true,\"font\":\"Lucida Sans\",\"fontColor\":\"black\",\"fontSize\":1.47,\"italicized\":false,\"underlined\":false},\"text\":\"EV (3)\",\"top\":627},\"label6287333563\":{\"deleted\":false,\"left\":126,\"settings\":{\"backgroundColor\":\"rgba(0, 0, 0, 0)\",\"bold\":true,\"font\":\"Lucida Sans\",\"fontColor\":\"black\",\"fontSize\":1.3,\"italicized\":false,\"underlined\":false},\"text\":\"Connection Duration\",\"top\":343},\"label7212972014\":{\"deleted\":false,\"left\":35,\"settings\":{\"backgroundColor\":\"rgba(0, 0, 0, 0)\",\"bold\":true,\"font\":\"Arial\",\"fontColor\":\"black\",\"fontSize\":2.6,\"italicized\":false,\"underlined\":false},\"text\":\"Simulation Settings\",\"top\":30},\"label7300068193\":{\"deleted\":false,\"left\":551,\"settings\":{\"backgroundColor\":\"rgba(0, 0, 0, 0)\",\"bold\":true,\"font\":\"Arial\",\"fontColor\":\"black\",\"fontSize\":1.47,\"italicized\":false,\"underlined\":false},\"text\":\"Initial SoC\",\"top\":491},\"label8610926686\":{\"deleted\":false,\"left\":889,\"settings\":{\"backgroundColor\":\"rgba(0, 0, 0, 0)\",\"bold\":true,\"font\":\"Arial\",\"fontColor\":\"black\",\"fontSize\":1.47,\"italicized\":false,\"underlined\":false},\"text\":\"Connection Duration\",\"top\":336},\"label9170590418\":{\"deleted\":false,\"left\":496,\"settings\":{\"backgroundColor\":\"rgba(0, 0, 0, 0)\",\"bold\":true,\"font\":\"Arial\",\"fontColor\":\"black\",\"fontSize\":1.47,\"italicized\":false,\"underlined\":false},\"text\":\"Connection Duration\",\"top\":341}},\"left\":344,\"name\":\"Panel\",\"panelId\":\"panelId-6772c4c8-0595-4f8c-93bd-17566f64b2d4\",\"tabIndex\":0,\"tabbedSetId\":\"tabbedSet1419519353\",\"top\":42,\"type\":\"panel\",\"version\":\"2019b\",\"visible\":false,\"width\":1252,\"zIndex\":1500012}"  PanelSnapshot=<binary blob, 63352 chars, not shown>  PanelBackground=data:image/png;base64,iVBORw0KGgoAAAANSUhEUgAABLsAAAMgCAYAAADLAGD1AAAABHNCSVQICAgIfAhkiAAAAAFzUkdCAK7OHOkAAAAEZ0FNQQAAsY8L/GEFAAAACXBIWXMAAA7EAAAOxAGVKw4bAAAAGXRFWHRTb2Z0d2FyZQB3d3cuaW5rc2NhcGUub3Jnm+48GgAAIwFJREFUeF7t3XuM5eVdx/Fn2OtAYemyWKViC7TQaqVV46XxEkt6oxdrJcWaGP8wxqrERK1WTaoUKG01KipivSQmjaZJSUytDa2mRG1rvNWqUArdlasIIswu12VmdnfOcc7wrN0uM7szZ36/M7/fZ16vZMP3WS677J/vfJ/nNzVcVAAAAAAgwCn1rwAAAADQe2IXAAAAADHELgAAAABiiF0A ...(+11764 chars)
